simulink model "UAV_modelo_naolinear_2"  (R2017a)
settings: Solver=ode45  StartTime=0.0  StopTime=T_sim  RelTol=1e-3  EnableMultiTasking=on
InitFcn:
  | main
values from neighbouring files (symbols this model uses):
  g = 9.8    [main_model1.m]    (also in main_model2.m; main_modelo_linear_v1.m; main_modelo_linear_v2.m; main_modelo_nao_linear_v1.m)
  incluir_din_motor = -1    [main_model1.m]    (also in main_model2.m; main_modelo_nao_linear_v1.m = 1; main_modelo_nao_linear_v2.m; modelo_naolinear.m = 1)
  Ir = 1e-3    (= 0.001)    [main_model1.m]    (also in main_model2.m; main_modelo_linear_v1.m = 0.01; main_modelo_linear_v2.m = 0.01; main_modelo_nao_linear_v1.m)
  Ixx = 1e-2    (= 0.01)    [main_model1.m]    (also in main_model2.m; main_modelo_linear_v1.m; main_modelo_linear_v2.m; main_modelo_nao_linear_v1.m)
  Iyy = 1e-2    (= 0.01)    [main_model1.m]    (also in main_model2.m; main_modelo_linear_v1.m; main_modelo_linear_v2.m; main_modelo_nao_linear_v1.m)
  Izz = 1.8e-2    (= 0.018)    [main_model1.m]    (also in main_model2.m; main_modelo_linear_v1.m; main_modelo_linear_v2.m; main_modelo_nao_linear_v1.m)
  K = are(A22, B22*inv(R)*B22',C'*Q*C)    [modelo_naolinear.m]    (also in modelo_naolinear_params.m)
  Kd_rot = 0.01    [main_model1.m]    (also in main_model2.m; main_modelo_linear_v1.m = 0; main_modelo_linear_v2.m = 0; main_modelo_nao_linear_v1.m)
  Kd_trans = 0.002    [main_model1.m]    (also in main_model2.m = -0.13723; main_modelo_linear_v1.m = 0; main_modelo_linear_v2.m = 0; main_modelo_nao_linear_v1.m)
  Ki_rot = 1.0    (= 1)    [main_model1.m]    (also in main_model2.m; main_modelo_linear_v1.m = 0.5; main_modelo_linear_v2.m = 0.5; main_modelo_nao_linear_v1.m)
  Ki_trans = 0.06    [main_model1.m]    (also in main_model2.m = 0.41774; main_modelo_linear_v1.m = 0; main_modelo_linear_v2.m = 1; main_modelo_nao_linear_v1.m)
  Kp = 0.9182    [main_model1.m]    (also in main_model2.m; main_modelo_nao_linear_v1.m; main_modelo_nao_linear_v2.m; modelo_naolinear.m)
  Kp_rot = 10    [main_model1.m]    (also in main_model2.m; main_modelo_linear_v1.m = 1; main_modelo_linear_v2.m = 1; main_modelo_nao_linear_v1.m)
  Kp_trans = 0.4    [main_model1.m]    (also in main_model2.m = 2.0968; main_modelo_linear_v1.m = 1; main_modelo_linear_v2.m = 2; main_modelo_nao_linear_v1.m)
  m = 1.0428    [main_model1.m]    (also in main_model2.m; main_modelo_linear_v1.m = 1; main_modelo_linear_v2.m = 1; main_modelo_nao_linear_v1.m)
  N_rot = 100    [main_model2.m]    (also in main_modelo_nao_linear_v2.m; modelo_naolinear.m; modelo_naolinear_params.m)
  N_trans = 5.5815    [main_model2.m]    (also in main_modelo_nao_linear_v2.m; modelo_naolinear.m; modelo_naolinear_params.m)
  p0 = 0    [main_model2.m]    (also in main_modelo_linear_v1.m; main_modelo_linear_v2.m; main_modelo_nao_linear_v2.m; modelo_naolinear.m)
  phi0 = 0    [main_model1.m]    (also in main_model2.m; main_modelo_linear_v1.m; main_modelo_linear_v2.m; main_modelo_nao_linear_v1.m)
  psi0 = 0    [main_model1.m]    (also in main_model2.m; main_modelo_linear_v1.m; main_modelo_linear_v2.m; main_modelo_nao_linear_v1.m)
  q0 = 0    [main_model2.m]    (also in main_modelo_linear_v1.m; main_modelo_linear_v2.m; main_modelo_nao_linear_v2.m; modelo_naolinear.m)
  r0 = 0    [main_model2.m]    (also in main_modelo_linear_v1.m; main_modelo_linear_v2.m; main_modelo_nao_linear_v2.m; modelo_naolinear.m)
  select_controlador = -1    [main_model2.m]    (also in main_modelo_nao_linear_v2.m)
  T = [kf,kf,kf,kf ... (first row only)    [main_model1.m]    (also in main_model2.m; main_modelo_nao_linear_v1.m; main_modelo_nao_linear_v2.m; modelo_naolinear.m)
  T_inv = T^(-1)    [main_model1.m]    (also in main_model2.m; main_modelo_nao_linear_v1.m; main_modelo_nao_linear_v2.m; modelo_naolinear.m)
  tau_a = 0.0569    [main_model1.m]    (also in main_model2.m; main_modelo_nao_linear_v1.m; main_modelo_nao_linear_v2.m; modelo_naolinear.m)
  tau_s = 0.0452    [main_model1.m]    (also in main_model2.m; main_modelo_nao_linear_v1.m; main_modelo_nao_linear_v2.m; modelo_naolinear.m)
  theta0 = 0    [main_model1.m]    (also in main_model2.m; main_modelo_linear_v1.m; main_modelo_linear_v2.m; main_modelo_nao_linear_v1.m)
  vx0 = 0    [main_model1.m]    (also in main_model2.m; main_modelo_nao_linear_v1.m; main_modelo_nao_linear_v2.m; modelo_naolinear.m)
  vxd = 0    [main_model1.m]    (also in main_model2.m; main_modelo_linear_v1.m; main_modelo_linear_v2.m; main_modelo_nao_linear_v1.m)
  vy0 = 0    [main_model1.m]    (also in main_model2.m; main_modelo_nao_linear_v1.m; main_modelo_nao_linear_v2.m; modelo_naolinear.m)
  vyd = 0    [main_model1.m]    (also in main_model2.m; main_modelo_linear_v1.m; main_modelo_linear_v2.m; main_modelo_nao_linear_v1.m)
  vz0 = 0    [main_model1.m]    (also in main_model2.m; main_modelo_nao_linear_v1.m; main_modelo_nao_linear_v2.m; modelo_naolinear.m)
  x0 = 0    [main_model1.m]    (also in main_model2.m; main_modelo_linear_v1.m; main_modelo_linear_v2.m; main_modelo_nao_linear_v1.m)
  y0 = 0    [main_model1.m]    (also in main_model2.m; main_modelo_linear_v1.m; main_modelo_linear_v2.m; main_modelo_nao_linear_v1.m)
  z0 = 1    [main_model1.m]    (also in main_model2.m; main_modelo_linear_v1.m; main_modelo_linear_v2.m; main_modelo_nao_linear_v1.m)
undefined symbols (not defined in the file or in its folder): sigbuilder_block
libraries: simulink x6
settings Model: Creator=dferr  LastModifiedBy=diego
settings DataIOCC: LimitDataPoints=on  SaveFormat=Array
settings OptimizationCC: LifeSpan=inf
settings DebuggingCC: SFUnexpectedBacktrackingDiag=warning  SFNoUnconditionalDefaultTransitionDiag=warning  SFExecutionAtInitializationDiag=none
settings HardwareCC: ProdBitPerPointer=32  ProdBitPerSizeT=32  ProdBitPerPtrDiffT=32  ProdLargestAtomicFloat=None  ProdIntDivRoundTo=Undefined  ProdEndianess=Unspecified  ProdWordSize=32  ProdHWDeviceType=32-bit Generic
settings ModelReferenceCC: PropagateSignalLabelsOutOfModel=off
settings GRTTargetCC: TargetLangStandard=C89/C90 (ANSI)  GeneratePreprocessorConditionals=Disable all
settings ConfigComp: CovMetricSettings=dw  CovHtmlReporting=on  CovSaveCumulativeToWorkspaceVar=on  CovSaveSingleToWorkspaceVar=on  CovExternalEMLEnable=off  CovSFcnEnable=off

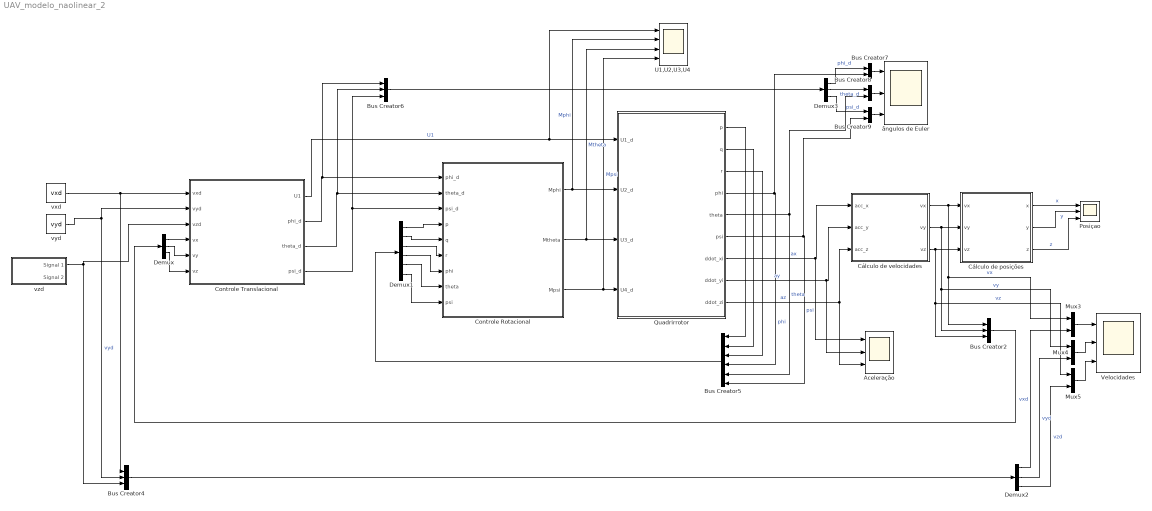
== system UAV_modelo_naolinear_2 ==
  Aceleração : Scope  NumInputPorts=3
  Bus Creator2 : BusCreator  Inputs=3
  Bus Creator4 : BusCreator  Inputs=3
  Bus Creator5 : BusCreator  Inputs=6
  Bus Creator6 : BusCreator  Inputs=3
  Bus Creator7 : BusCreator  Inputs=2
  Bus Creator8 : BusCreator  Inputs=2
  Bus Creator9 : BusCreator  Inputs=2
  Controle Rotacional : Subsystem
      mask Display:
      | disp('Controle Rotacional')
      | port_label('input',1,'phi_d')
      | port_label('input',2,'theta_d')
      | port_label('input',3,'psi_d')
      | port_label('input',4,'p')
      | port_label('input',5,'q')
      | port_label('input',6,'r')
      | port_label('input',7,'phi')
      | port_label('input',8,'theta')
      | port_label('input',9,'psi')
      | port_label('output',1,'Mphi')
      | port_label('output',2,'Mtheta')
      | port_label('output',3,'Mpsi')
  Controle Translacional : Subsystem
      mask Display:
      | disp('Controle Translacional')
      | port_label('input',1,'vxd')
      | port_label('input',2,'vyd')
      | port_label('input',3,'vzd')
      | port_label('input',4,'vx')
      | port_label('input',5,'vy')
      | port_label('input',6,'vz')
      | port_label('output',1,'U1')
      | port_label('output',2,'phi_d')
      | port_label('output',3,'theta_d')
      | port_label('output',4,'psi_d')
  Cálculo de posições : Subsystem
      mask Display:
      | disp('Vel -> Pos')
      | port_label('input',1,'vel_x')
      | port_label('input',2,'vel_y')
      | port_label('input',3,'vel_ z')
      | port_label('output',1,'x')
      | port_label('output',2,'y')
      | port_label('output',3,'z')
  Cálculo de velocidades : Subsystem
      mask Display:
      | disp('Acc -> Vel')
      | port_label('input',1,'acc_x')
      | port_label('input',2,'acc_y')
      | port_label('input',3,'acc_z')
      | port_label('output',1,'vel_x')
      | port_label('output',2,'vel_y')
      | port_label('output',3,'vel_z')
  Demux : Demux  Outputs=3
  Demux1 : Demux  Outputs=6
  Demux2 : Demux  Outputs=3
  Demux3 : Demux  Outputs=3
  Mux3 : Mux  Inputs=2
  Mux4 : Mux  Inputs=2
  Mux5 : Mux  Inputs=2
  Posiçao : Scope  NumInputPorts=3
  Quadrirrotor : Subsystem
      mask Display:
      | disp('Quadrirrotor')
      | port_label('input',1,'U1')
      | port_label('input',2,'U2')
      | port_label('input',3,'U3')
      | port_label('input',4,'U4')
      | port_label('output',1,'p')
      | port_label('output',2,'q')
      | port_label('output',3,'r')
      | port_label('output',4,'phi')
      | port_label('output',5,'theta')
      | port_label('output',6,'psi')
      | port_label('output',7,'ddot_xi')
      | port_label('output',8,'ddot_yi')
      | port_label('output',9,'ddot_zi')
  U1,U2,U3,U4 : Scope  NumInputPorts=4
  Velocidades : Scope  NumInputPorts=3
  vxd : Constant  Value=vxd
  vyd : Constant  Value=vyd
  vzd : Subsystem  Tag=STV Subsys  LoadFcn=sigbuilder_block('load');  StartFcn=sigbuilder_block('start');  StopFcn=sigbuilder_block('stop');  ClipboardFcn=sigbuilder_block('clipboard');  mask(Sigbuilder block){tuvar=[0:10]}
      mask help: Simulink:masks:SigbuilderBlock_MD
      mask init:
      | if ~strcmp(get_param(bdroot(gcbh),'SimulationStatus'),'stopped') tuvar = sigbuilder_block('maskInit'); end
      settings: CopyFcn=sigbuilder_block('copy');  DeleteFcn=sigbuilder_block('delete');  ModelCloseFcn=sigbuilder_block('modelClose');  PreSaveFcn=sigbuilder_block('preSave');  PauseFcn=sigbuilder_block('pause');  ContinueFcn=sigbuilder_block('continue');  NameChangeFcn=sigbuilder_block('namechange');  OpenFcn=sigbuilder_block('open',[437.6 199.2 550.4 400 ]);  CloseFcn=sigbuilder_block('close');
      mask Display: plot(0, 0, 100, 100,[2, 2, 32, 32, 2], [68, 8, 8, 68, 68],[32, 2], [38, 38], [32, 19, 2],[53, 60, 44], [32, 17, 17, 2],[16, 16, 31, 31]);txt = getActiveGroup(gcbh);text(2, 100, txt,'verticalAlignment', 'top');
  ângulos de Euler : Scope  NumInputPorts=3
  wires:
  Cálculo de velocidades/1(vx) -> Mux3/1, Bus Creator2/1, Cálculo de posições/1(vx)  "vx"
  Cálculo de velocidades/2(vy) -> Mux4/1, Bus Creator2/2, Cálculo de posições/2(vy)  "vy"
  Cálculo de velocidades/3(vz) -> Mux5/1, Bus Creator2/3, Cálculo de posições/3(vz)  "vz"
  Bus Creator2/1 -> Demux/1
  vyd/1 -> Controle Translacional/2(vyd), Bus Creator4/2  "vyd"
  Demux1/1 -> Controle Rotacional/4(p)
  Demux1/2 -> Controle Rotacional/5(q)
  Demux1/3 -> Controle Rotacional/6(r)
  Demux1/4 -> Controle Rotacional/7(phi)
  Demux1/5 -> Controle Rotacional/8(theta)
  Demux1/6 -> Controle Rotacional/9(psi)
  Bus Creator5/1 -> Demux1/1
  Mux3/1 -> Velocidades/1
  Mux4/1 -> Velocidades/2
  Mux5/1 -> Velocidades/3
  Bus Creator4/1 -> Demux2/1
  Demux2/1 -> Mux3/2  "vxd"
  Demux2/2 -> Mux4/2  "vyd"
  Demux2/3 -> Mux5/2  "vzd"
  Controle Rotacional/1(Mphi) -> U1,U2,U3,U4/2, Quadrirrotor/2(U2_d)  "Mphi"
  Controle Rotacional/2(Mtheta) -> U1,U2,U3,U4/3, Quadrirrotor/3(U3_d)  "Mtheta"
  Controle Rotacional/3(Mpsi) -> U1,U2,U3,U4/4, Quadrirrotor/4(U4_d)  "Mpsi"
  Quadrirrotor/1(p) -> Bus Creator5/1
  Quadrirrotor/2(q) -> Bus Creator5/2
  Quadrirrotor/3(r) -> Bus Creator5/3
  Quadrirrotor/4(phi) -> Bus Creator7/2, Bus Creator5/4  "phi"
  Quadrirrotor/5(theta) -> Bus Creator5/5, Bus Creator8/2  "theta"
  Quadrirrotor/6(psi) -> Bus Creator9/2, Bus Creator5/6  "psi"
  Quadrirrotor/7(ddot_xi) -> Aceleração/1, Cálculo de velocidades/1(acc_x)  "ax"
  Quadrirrotor/8(ddot_yi) -> Aceleração/2, Cálculo de velocidades/2(acc_y)  "ay"
  Quadrirrotor/9(ddot_zi) -> Aceleração/3, Cálculo de velocidades/3(acc_z)  "az"
  Demux/1 -> Controle Translacional/4(vx)
  Demux/2 -> Controle Translacional/5(vy)
  Demux/3 -> Controle Translacional/6(vz)
  Controle Translacional/1(U1) -> U1,U2,U3,U4/1, Quadrirrotor/1(U1_d)  "U1"
  Controle Translacional/2(phi_d) -> Bus Creator6/1, Controle Rotacional/1(phi_d)
  Controle Translacional/3(theta_d) -> Bus Creator6/2, Controle Rotacional/2(theta_d)
  Controle Translacional/4(psi_d) -> Bus Creator6/3, Controle Rotacional/3(psi_d)
  Bus Creator6/1 -> Demux3/1
  Bus Creator7/1 -> ângulos de Euler/1
  Bus Creator8/1 -> ângulos de Euler/2
  Bus Creator9/1 -> ângulos de Euler/3
  Demux3/1 -> Bus Creator7/1  "phi_d"
  Demux3/2 -> Bus Creator8/1  "theta_d"
  Demux3/3 -> Bus Creator9/1  "psi_d"
  vxd/1 -> Bus Creator4/1, Controle Translacional/1(vxd)
  Cálculo de posições/1(x) -> Posiçao/1  "x"
  Cálculo de posições/2(y) -> Posiçao/2  "y"
  Cálculo de posições/3(z) -> Posiçao/3  "z"
  vzd/1(Signal 1) -> Controle Translacional/3(vzd), Bus Creator4/3

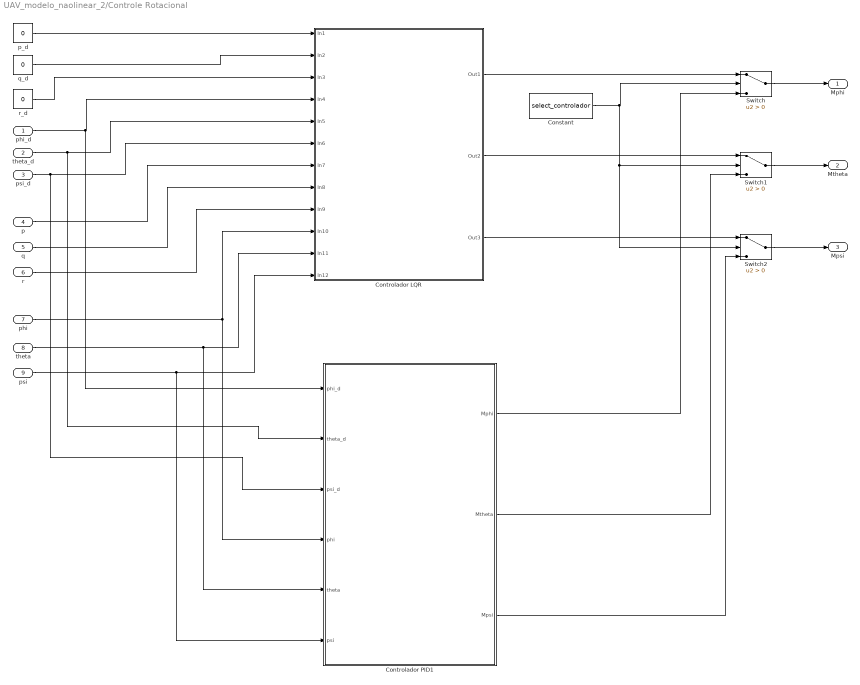
== system UAV_modelo_naolinear_2/Controle Rotacional ==
  phi_d : Inport
  theta_d : Inport  Port=2
  psi_d : Inport  Port=3
  p : Inport  Port=4
  q : Inport  Port=5
  r : Inport  Port=6
  phi : Inport  Port=7
  theta : Inport  Port=8
  psi : Inport  Port=9
  Constant : Constant  Value=select_controlador
  Controlador LQR : Subsystem
      mask Display:
      | disp('Controlador LQR')
      | port_label('input',1,'p_d')
      | port_label('input',2,'q_d')
      | port_label('input',3,'r_d')
      | port_label('input',4,'phi_d')
      | port_label('input',5,'theta_d')
      | port_label('input',6,'psi_d')
      | port_label('input',7,'p')
      | port_label('input',8,'q')
      | port_label('input',9,'r')
      | port_label('input',10,'phi')
      | port_label('input',11,'theta')
      | port_label('input',12,'psi')
      | port_label('output',1,'Mphi')
      | port_label('output',2,'Mtheta')
      | port_label('output',3,'Mpsi')
  Controlador PID1 : Subsystem
      mask Display:
      | disp('Controlador PID')
      | port_label('input',1,'phi_d')
      | port_label('input',2,'theta_d')
      | port_label('input',3,'psi_d')
      | port_label('input',4,'phi')
      | port_label('input',5,'theta')
      | port_label('input',6,'psi')
      | port_label('output',1,'Mphi')
      | port_label('output',2,'Mtheta')
      | port_label('output',3,'Mpsi')
  Switch : Switch  Criteria=u2 > Threshold
  Switch1 : Switch  Criteria=u2 > Threshold
  Switch2 : Switch  Criteria=u2 > Threshold
  p_d : Constant  Value=0
  q_d : Constant  Value=0
  r_d : Constant  Value=0
  Mphi : Outport
  Mtheta : Outport  Port=2
  Mpsi : Outport  Port=3
  wires:
  p_d/1 -> Controlador LQR/1(In1)
  q_d/1 -> Controlador LQR/2(In2)
  r_d/1 -> Controlador LQR/3(In3)
  phi_d/1 -> Controlador PID1/1(phi_d), Controlador LQR/4(In4)
  theta_d/1 -> Controlador PID1/2(theta_d), Controlador LQR/5(In5)
  psi_d/1 -> Controlador PID1/3(psi_d), Controlador LQR/6(In6)
  p/1 -> Controlador LQR/7(In7)
  q/1 -> Controlador LQR/8(In8)
  r/1 -> Controlador LQR/9(In9)
  phi/1 -> Controlador PID1/4(phi), Controlador LQR/10(In10)
  theta/1 -> Controlador PID1/5(theta), Controlador LQR/11(In11)
  psi/1 -> Controlador PID1/6(psi), Controlador LQR/12(In12)
  Controlador LQR/1(Out1) -> Switch/1
  Controlador LQR/3(Out3) -> Switch2/1
  Controlador LQR/2(Out2) -> Switch1/1
  Switch/1 -> Mphi/1
  Switch1/1 -> Mtheta/1
  Switch2/1 -> Mpsi/1
  Constant/1 -> Switch2/2, Switch1/2, Switch/2
  Controlador PID1/1(Mphi) -> Switch/3
  Controlador PID1/2(Mtheta) -> Switch1/3
  Controlador PID1/3(Mpsi) -> Switch2/3

== system UAV_modelo_naolinear_2/Controle Translacional ==
  vxd : Inport
  vyd : Inport  Port=2
  vzd : Inport  Port=3
  vx : Inport  Port=4
  vy : Inport  Port=5
  vz : Inport  Port=6
  Controle de velocidade : Subsystem
      mask Display:
      | disp('Controle de Velocidade PID')
      | port_label('input',1,'vxd')
      | port_label('input',2,'vyd')
      | port_label('input',3,'vzd')
      | port_label('input',4,'vx')
      | port_label('input',5,'vy')
      | port_label('input',6,'vz')
      | 
      | port_label('output',1,'u1')
      | port_label('output',2,'u2')
      | port_label('output',3,'u3')
  Entradas virtuais : Subsystem
      mask Display:
      | disp('(u1,u2,u3)->(eta_d,U1)')
      | port_label('input',1,'u1')
      | port_label('input',2,'u2')
      | port_label('input',3,'u3')
      | port_label('output',1,'phi_d')
      | port_label('output',2,'theta_d')
      | port_label('output',3,'psi_d')
      | port_label('output',4,'U1')
  U1 : Outport
  phi_d : Outport  Port=2
  theta_d : Outport  Port=3
  psi_d : Outport  Port=4
  wires:
  Controle de velocidade/2(u2) -> Entradas virtuais/2(u2)
  Entradas virtuais/1(phi_d) -> phi_d/1  "phi_d"
  Entradas virtuais/2(theta_d) -> theta_d/1  "theta_d"
  Entradas virtuais/3(psi_d) -> psi_d/1  "psi_d"
  Controle de velocidade/1(u1) -> Entradas virtuais/1(u1)
  vz/1 -> Controle de velocidade/6(vz)
  vy/1 -> Controle de velocidade/5("vy ")
  Controle de velocidade/3(u3) -> Entradas virtuais/3(u3)
  vx/1 -> Controle de velocidade/4(vx)
  Entradas virtuais/4(U1) -> U1/1  "Tb"
  vyd/1 -> Controle de velocidade/2(vyd)
  vzd/1 -> Controle de velocidade/3(vzd)
  vxd/1 -> Controle de velocidade/1(vxd)

== system UAV_modelo_naolinear_2/Cálculo de posições ==
  vx : Inport
  vy : Inport  Port=2
  vz : Inport  Port=3
  Integrator : Integrator  InitialCondition=x0
  Integrator1 : Integrator  InitialCondition=y0
  Integrator2 : Integrator  InitialCondition=z0  LimitOutput=on  LowerSaturationLimit=0
  x : Outport
  y : Outport  Port=2
  z : Outport  Port=3
  wires:
  Integrator/1 -> x/1
  Integrator1/1 -> y/1
  vy/1 -> Integrator1/1
  vz/1 -> Integrator2/1
  vx/1 -> Integrator/1
  Integrator2/1 -> z/1

== system UAV_modelo_naolinear_2/Cálculo de velocidades ==
  acc_x : Inport
  acc_y : Inport  Port=2
  acc_z : Inport  Port=3
  Integrator : Integrator  InitialCondition=vx0  ZeroCross=off
  Integrator1 : Integrator  InitialCondition=vy0  ZeroCross=off
  Integrator2 : Integrator  InitialCondition=vz0  ZeroCross=off
  vx : Outport
  vy : Outport  Port=2
  vz : Outport  Port=3
  wires:
  Integrator2/1 -> vz/1
  acc_z/1 -> Integrator2/1
  Integrator/1 -> vx/1
  acc_x/1 -> Integrator/1
  acc_y/1 -> Integrator1/1
  Integrator1/1 -> vy/1

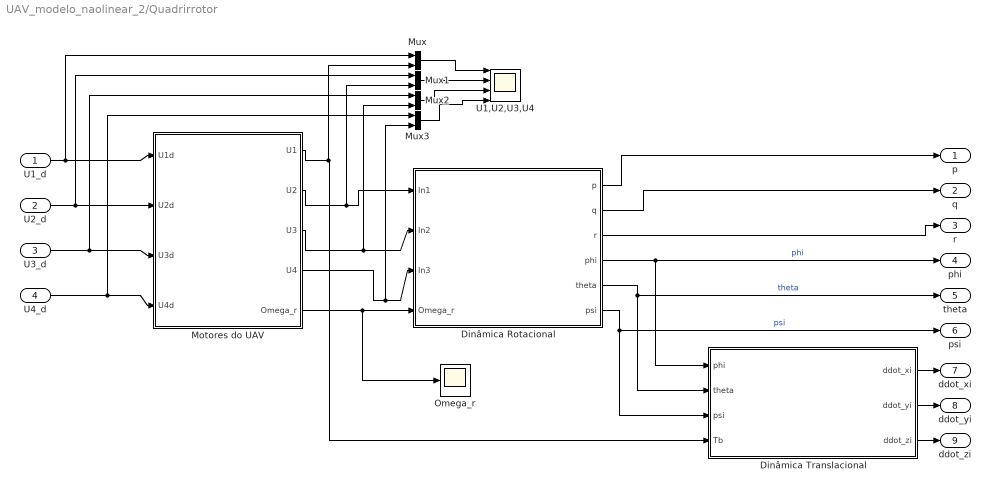
== system UAV_modelo_naolinear_2/Quadrirrotor ==
  U1_d : Inport
  U2_d : Inport  Port=2
  U3_d : Inport  Port=3
  U4_d : Inport  Port=4
  Dinâmica Rotacional : Subsystem
      mask Display:
      | disp('Dinâmica Rotacional')
      | port_label('input',1,'Mphi')
      | port_label('input',2,'Mtheta')
      | port_label('input',3,'Mpsi')
      | port_label('input',4,'Omega_r')
      | port_label('output',1,'p')
      | port_label('output',2,'q')
      | port_label('output',3,'r')
      | port_label('output',4,'phi')
      | port_label('output',5,'theta')
      | port_label('output',6,'psi')
  Dinâmica Translacional : Subsystem
      mask Display:
      | disp ('Dinâmica Translacional')
      | port_label('input',1,'phi')
      | port_label('input',2,'theta')
      | port_label('input',3,'psi')
      | port_label('input',4,'Tb')
      | port_label('output',1,'ddot_xi')
      | port_label('output',2,'ddot_yi')
      | port_label('output',3,'ddot_zi')
  "Motores do UAV " : Subsystem
      mask Display:
      | disp('Dinâmica Motores')
      | port_label('input',1,'U1d')
      | port_label('input',2,'U2d')
      | port_label('input',3,'U3d')
      | port_label('input',4,'U4d')
      | port_label('output',1,'U1')
      | port_label('output',2,'U2')
      | port_label('output',3,'U3')
      | port_label('output',4,'U4')
      | port_label('output',5,'Omega_r')
  Mux{,1..3} (4 alike) : Mux  Inputs=2
  Omega_r : Scope
  U1,U2,U3,U4 : Scope  NumInputPorts=4
  p : Outport
  q : Outport  Port=2
  r : Outport  Port=3
  phi : Outport  Port=4
  theta : Outport  Port=5
  psi : Outport  Port=6
  ddot_xi : Outport  Port=7
  ddot_yi : Outport  Port=8
  ddot_zi : Outport  Port=9
  wires:
  Dinâmica Rotacional/6(psi) -> psi/1, Dinâmica Translacional/3(psi)  "psi"
  Dinâmica Rotacional/5(theta) -> theta/1, Dinâmica Translacional/2(theta)  "theta"
  Dinâmica Rotacional/4(phi) -> Dinâmica Translacional/1(phi), phi/1  "phi"
  Dinâmica Rotacional/1(p) -> p/1
  Dinâmica Rotacional/2(q) -> q/1
  Dinâmica Rotacional/3(r) -> r/1
  Dinâmica Translacional/1(ddot_xi) -> ddot_xi/1
  Dinâmica Translacional/2(ddot_yi) -> ddot_yi/1
  Dinâmica Translacional/3(ddot_zi) -> ddot_zi/1
  U2_d/1 -> "Motores do UAV "/2(U2d), Mux1/1
  U3_d/1 -> "Motores do UAV "/3(U3d), Mux2/1
  Mux/1 -> U1,U2,U3,U4/1
  Mux1/1 -> U1,U2,U3,U4/2
  Mux2/1 -> U1,U2,U3,U4/3
  Mux3/1 -> U1,U2,U3,U4/4
  "Motores do UAV "/3(U3) -> Mux2/2, Dinâmica Rotacional/2(In2)
  "Motores do UAV "/4(U4) -> Mux3/2, Dinâmica Rotacional/3(In3)
  "Motores do UAV "/2(U2) -> Mux1/2, Dinâmica Rotacional/1(In1)
  "Motores do UAV "/1(U1) -> Mux/2, Dinâmica Translacional/4(Tb)
  U1_d/1 -> "Motores do UAV "/1(U1d), Mux/1
  U4_d/1 -> "Motores do UAV "/4(U4d), Mux3/1
  "Motores do UAV "/5(Omega_r) -> Omega_r/1, Dinâmica Rotacional/4(Omega_r)

== system UAV_modelo_naolinear_2/vzd ==
  Demux : Demux  Tag=STV Demux  Outputs=2
  FromWs : FromWorkspace  Tag=STV FromWs  VariableName=tuvar  SampleTime=0
      SigBuilderData=|
      | common.afterFinalStr = 'Extrapolate'
      | common.sampleTime = 0
      | dataSet.timeRange = [0 20]
      | dataSet.name = 'Group 1'
      | sbobj.Groups.Name = 'Group 1'
      | sbobj.Groups.Signals(1).Name = 'Signal 1'
      | sbobj.Groups.Signals(1).XData = [0 2.05 4.75 8 18 20]
      | sbobj.Groups.Signals(1).YData = [-0.2 8.5 20 20 0 0]
      | sbobj.Groups.Signals(2).Name = 'Signal 2'
      | sbobj.Groups.Signals(2).XData = [0 5 5 20]
      | sbobj.Groups.Signals(2).YData = [0 0 1 1]
      | sbobj.Groups.TimeRange = [0 20]
  Signal 1 : Outport  Tag=STV Outport
  Signal 2 : Outport  Tag=STV Outport  Port=2
  wires:
  FromWs/1 -> Demux/1
  Demux/1 -> Signal 1/1
  Demux/2 -> Signal 2/1

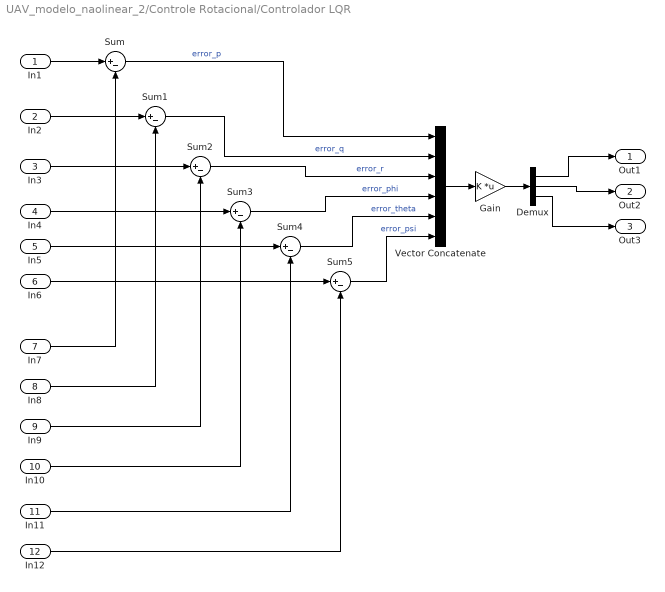
== system UAV_modelo_naolinear_2/Controle Rotacional/Controlador LQR ==
  In1 : Inport
  In2 : Inport  Port=2
  In3 : Inport  Port=3
  In4 : Inport  Port=4
  In5 : Inport  Port=5
  In6 : Inport  Port=6
  In7 : Inport  Port=7
  In8 : Inport  Port=8
  In9 : Inport  Port=9
  In10 : Inport  Port=10
  In11 : Inport  Port=11
  In12 : Inport  Port=12
  Demux : Demux  Outputs=3
  Gain : Gain  Gain=K  Multiplication=Matrix(K*u)
  Sum{,1..5} (6 alike) : Sum  Inputs=|+-
  Vector Concatenate : Concatenate  NumInputs=6
  Out1 : Outport
  Out2 : Outport  Port=2
  Out3 : Outport  Port=3
  wires:
  In3/1 -> Sum2/1
  Sum4/1 -> Vector Concatenate/5  "error_theta"
  Gain/1 -> Demux/1
  Demux/2 -> Out2/1
  In5/1 -> Sum4/1
  In11/1 -> Sum4/2
  Demux/3 -> Out3/1
  In4/1 -> Sum3/1
  Vector Concatenate/1 -> Gain/1
  Sum5/1 -> Vector Concatenate/6  "error_psi"
  In8/1 -> Sum1/2
  In2/1 -> Sum1/1
  In1/1 -> Sum/1
  In12/1 -> Sum5/2
  In9/1 -> Sum2/2
  Demux/1 -> Out1/1
  Sum2/1 -> Vector Concatenate/3  "error_r"
  In6/1 -> Sum5/1
  In7/1 -> Sum/2
  In10/1 -> Sum3/2
  Sum/1 -> Vector Concatenate/1  "error_p"
  Sum1/1 -> Vector Concatenate/2  "error_q"
  Sum3/1 -> Vector Concatenate/4  "error_phi"

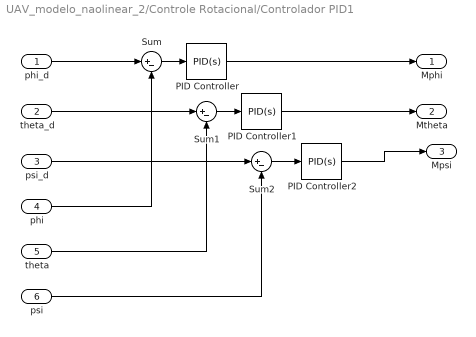
== system UAV_modelo_naolinear_2/Controle Rotacional/Controlador PID1 ==
  phi_d : Inport
  theta_d : Inport  Port=2
  psi_d : Inport  Port=3
  phi : Inport  Port=4
  theta : Inport  Port=5
  psi : Inport  Port=6
  PID Controller : simulink/Continuous/PID Controller  Controller=PID  TimeDomain=Continuous-time  SampleTime=-1  IntegratorMethod=Forward Euler  FilterMethod=Forward Euler  Form=Ideal  UseFilter=on  ControllerParametersSource=internal  P=Kp_rot  I=Ki_rot  D=Kd_rot  N=N_rot  InitialConditionSource=internal  InitialConditionForIntegrator=0  InitialConditionForFilter=0  ExternalReset=none  LimitOutput=off  UpperSaturationLimit=inf  LowerSaturationLimit=-inf  LinearizeAsGain=on  AntiWindupMode=none  Kb=1  TrackingMode=off  Kt=1  PParamMin=[]  PParamMax=[]  IParamMin=[]  IParamMax=[]  DParamMin=[]  DParamMax=[]  NParamMin=[]  NParamMax=[]  KbParamMin=[]  KbParamMax=[]  KtParamMin=[]  KtParamMax=[]  POutMin=[]  POutMax=[]  IOutMin=[]  IOutMax=[]  DOutMin=[]  DOutMax=[]  NOutMin=[]  NOutMax=[]  KbOutMin=[]  KbOutMax=[]  KtOutMin=[]  KtOutMax=[]  IntegratorOutMin=[]  IntegratorOutMax=[]  FilterOutMin=[]  FilterOutMax=[]  SumOutMin=[]  SumOutMax=[]  SumI1OutMin=[]  SumI1OutMax=[]  SumI2OutMin=[]  SumI2OutMax=[]  SumI3OutMin=[]  SumI3OutMax=[]  SumDOutMin=[]  SumDOutMax=[]  SaturationOutMin=[]  SaturationOutMax=[]  IntegratorContinuousStateAttributes=''  IntegratorStateMustResolveToSignalObject=off  IntegratorRTWStateStorageClass=Auto  FilterContinuousStateAttributes=''  FilterStateMustResolveToSignalObject=off  FilterRTWStateStorageClass=Auto  DifferentiatorICPrevScaledInput=0  DifferentiatorOutMin=[]  DifferentiatorOutMax=[]  InitialConditionSetting=State (most efficient)
  PID Controller1 : simulink/Continuous/PID Controller  Controller=PID  TimeDomain=Continuous-time  SampleTime=-1  IntegratorMethod=Forward Euler  FilterMethod=Forward Euler  Form=Ideal  UseFilter=on  ControllerParametersSource=internal  P=Kp_rot  I=Ki_rot  D=Kd_rot  N=N_rot  InitialConditionSource=internal  InitialConditionForIntegrator=0  InitialConditionForFilter=0  ExternalReset=none  LimitOutput=off  UpperSaturationLimit=inf  LowerSaturationLimit=-inf  LinearizeAsGain=on  AntiWindupMode=none  Kb=1  TrackingMode=off  Kt=1  PParamMin=[]  PParamMax=[]  IParamMin=[]  IParamMax=[]  DParamMin=[]  DParamMax=[]  NParamMin=[]  NParamMax=[]  KbParamMin=[]  KbParamMax=[]  KtParamMin=[]  KtParamMax=[]  POutMin=[]  POutMax=[]  IOutMin=[]  IOutMax=[]  DOutMin=[]  DOutMax=[]  NOutMin=[]  NOutMax=[]  KbOutMin=[]  KbOutMax=[]  KtOutMin=[]  KtOutMax=[]  IntegratorOutMin=[]  IntegratorOutMax=[]  FilterOutMin=[]  FilterOutMax=[]  SumOutMin=[]  SumOutMax=[]  SumI1OutMin=[]  SumI1OutMax=[]  SumI2OutMin=[]  SumI2OutMax=[]  SumI3OutMin=[]  SumI3OutMax=[]  SumDOutMin=[]  SumDOutMax=[]  SaturationOutMin=[]  SaturationOutMax=[]  IntegratorContinuousStateAttributes=''  IntegratorStateMustResolveToSignalObject=off  IntegratorRTWStateStorageClass=Auto  FilterContinuousStateAttributes=''  FilterStateMustResolveToSignalObject=off  FilterRTWStateStorageClass=Auto  DifferentiatorICPrevScaledInput=0  DifferentiatorOutMin=[]  DifferentiatorOutMax=[]  InitialConditionSetting=State (most efficient)
  PID Controller2 : simulink/Continuous/PID Controller  Controller=PID  TimeDomain=Continuous-time  SampleTime=-1  IntegratorMethod=Forward Euler  FilterMethod=Forward Euler  Form=Ideal  UseFilter=on  ControllerParametersSource=internal  P=Kp_rot  I=Ki_rot  D=Kd_rot  N=N_rot  InitialConditionSource=internal  InitialConditionForIntegrator=0  InitialConditionForFilter=0  ExternalReset=none  LimitOutput=off  UpperSaturationLimit=inf  LowerSaturationLimit=-inf  LinearizeAsGain=on  AntiWindupMode=none  Kb=1  TrackingMode=off  Kt=1  PParamMin=[]  PParamMax=[]  IParamMin=[]  IParamMax=[]  DParamMin=[]  DParamMax=[]  NParamMin=[]  NParamMax=[]  KbParamMin=[]  KbParamMax=[]  KtParamMin=[]  KtParamMax=[]  POutMin=[]  POutMax=[]  IOutMin=[]  IOutMax=[]  DOutMin=[]  DOutMax=[]  NOutMin=[]  NOutMax=[]  KbOutMin=[]  KbOutMax=[]  KtOutMin=[]  KtOutMax=[]  IntegratorOutMin=[]  IntegratorOutMax=[]  FilterOutMin=[]  FilterOutMax=[]  SumOutMin=[]  SumOutMax=[]  SumI1OutMin=[]  SumI1OutMax=[]  SumI2OutMin=[]  SumI2OutMax=[]  SumI3OutMin=[]  SumI3OutMax=[]  SumDOutMin=[]  SumDOutMax=[]  SaturationOutMin=[]  SaturationOutMax=[]  IntegratorContinuousStateAttributes=''  IntegratorStateMustResolveToSignalObject=off  IntegratorRTWStateStorageClass=Auto  FilterContinuousStateAttributes=''  FilterStateMustResolveToSignalObject=off  FilterRTWStateStorageClass=Auto  DifferentiatorICPrevScaledInput=0  DifferentiatorOutMin=[]  DifferentiatorOutMax=[]  InitialConditionSetting=State (most efficient)
  Sum : Sum  Inputs=|+-
  Sum1 : Sum  Inputs=|+-
  Sum2 : Sum  Inputs=|+-
  Mphi : Outport
  Mtheta : Outport  Port=2
  Mpsi : Outport  Port=3
  wires:
  PID Controller2/1 -> Mpsi/1
  PID Controller1/1 -> Mtheta/1
  PID Controller/1 -> Mphi/1
  Sum/1 -> PID Controller/1
  Sum1/1 -> PID Controller1/1
  Sum2/1 -> PID Controller2/1
  phi_d/1 -> Sum/1
  theta_d/1 -> Sum1/1
  psi_d/1 -> Sum2/1
  phi/1 -> Sum/2
  theta/1 -> Sum1/2
  psi/1 -> Sum2/2

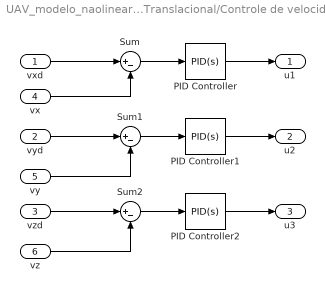
== system UAV_modelo_naolinear_2/Controle Translacional/Controle de velocidade ==
  vxd : Inport
  vyd : Inport  Port=2
  vzd : Inport  Port=3
  vx : Inport  Port=4
  "vy " : Inport  Port=5
  vz : Inport  Port=6
  PID Controller : simulink/Continuous/PID Controller  Controller=PID  TimeDomain=Continuous-time  SampleTime=-1  IntegratorMethod=Forward Euler  FilterMethod=Forward Euler  Form=Parallel  UseFilter=on  ControllerParametersSource=internal  P=Kp_trans  I=Ki_trans  D=Kd_trans  N=N_trans  InitialConditionSource=internal  InitialConditionForIntegrator=0  InitialConditionForFilter=0  ExternalReset=none  LimitOutput=off  UpperSaturationLimit=inf  LowerSaturationLimit=-inf  LinearizeAsGain=on  AntiWindupMode=none  Kb=1  TrackingMode=off  Kt=1  RndMeth=Nearest  PParamMin=[]  PParamMax=[]  IParamMin=[]  IParamMax=[]  DParamMin=[]  DParamMax=[]  NParamMin=[]  NParamMax=[]  KbParamMin=[]  KbParamMax=[]  KtParamMin=[]  KtParamMax=[]  POutMin=[]  POutMax=[]  IOutMin=[]  IOutMax=[]  DOutMin=[]  DOutMax=[]  NOutMin=[]  NOutMax=[]  KbOutMin=[]  KbOutMax=[]  KtOutMin=[]  KtOutMax=[]  IntegratorOutMin=[]  IntegratorOutMax=[]  FilterOutMin=[]  FilterOutMax=[]  SumOutMin=[]  SumOutMax=[]  SumI1OutMin=[]  SumI1OutMax=[]  SumI2OutMin=[]  SumI2OutMax=[]  SumI3OutMin=[]  SumI3OutMax=[]  SumDOutMin=[]  SumDOutMax=[]  SaturationOutMin=[]  SaturationOutMax=[]  IntegratorContinuousStateAttributes=''  IntegratorStateMustResolveToSignalObject=off  IntegratorRTWStateStorageClass=Auto  FilterContinuousStateAttributes=''  FilterStateMustResolveToSignalObject=off  FilterRTWStateStorageClass=Auto  DifferentiatorICPrevScaledInput=0  DifferentiatorOutMin=[]  DifferentiatorOutMax=[]  InitialConditionSetting=State (most efficient)
      settings: LockScale=on
  PID Controller1 : simulink/Continuous/PID Controller  Controller=PID  TimeDomain=Continuous-time  SampleTime=-1  IntegratorMethod=Forward Euler  FilterMethod=Forward Euler  Form=Parallel  UseFilter=on  ControllerParametersSource=internal  P=Kp_trans  I=Ki_trans  D=Kd_trans  N=100  InitialConditionSource=internal  InitialConditionForIntegrator=0  InitialConditionForFilter=0  ExternalReset=none  LimitOutput=off  UpperSaturationLimit=inf  LowerSaturationLimit=-inf  LinearizeAsGain=on  AntiWindupMode=none  Kb=1  TrackingMode=off  Kt=1  RndMeth=Nearest  PParamMin=[]  PParamMax=[]  IParamMin=[]  IParamMax=[]  DParamMin=[]  DParamMax=[]  NParamMin=[]  NParamMax=[]  KbParamMin=[]  KbParamMax=[]  KtParamMin=[]  KtParamMax=[]  POutMin=[]  POutMax=[]  IOutMin=[]  IOutMax=[]  DOutMin=[]  DOutMax=[]  NOutMin=[]  NOutMax=[]  KbOutMin=[]  KbOutMax=[]  KtOutMin=[]  KtOutMax=[]  IntegratorOutMin=[]  IntegratorOutMax=[]  FilterOutMin=[]  FilterOutMax=[]  SumOutMin=[]  SumOutMax=[]  SumI1OutMin=[]  SumI1OutMax=[]  SumI2OutMin=[]  SumI2OutMax=[]  SumI3OutMin=[]  SumI3OutMax=[]  SumDOutMin=[]  SumDOutMax=[]  SaturationOutMin=[]  SaturationOutMax=[]  IntegratorContinuousStateAttributes=''  IntegratorStateMustResolveToSignalObject=off  IntegratorRTWStateStorageClass=Auto  FilterContinuousStateAttributes=''  FilterStateMustResolveToSignalObject=off  FilterRTWStateStorageClass=Auto  DifferentiatorICPrevScaledInput=0  DifferentiatorOutMin=[]  DifferentiatorOutMax=[]  InitialConditionSetting=State (most efficient)
      settings: LockScale=on
  PID Controller2 : simulink/Continuous/PID Controller  Controller=PID  TimeDomain=Continuous-time  SampleTime=-1  IntegratorMethod=Forward Euler  FilterMethod=Forward Euler  Form=Parallel  UseFilter=on  ControllerParametersSource=internal  P=Kp_trans  I=Ki_trans  D=Kd_trans  N=100  InitialConditionSource=internal  InitialConditionForIntegrator=0  InitialConditionForFilter=0  ExternalReset=none  LimitOutput=off  UpperSaturationLimit=inf  LowerSaturationLimit=-inf  LinearizeAsGain=on  AntiWindupMode=none  Kb=1  TrackingMode=off  Kt=1  RndMeth=Nearest  PParamMin=[]  PParamMax=[]  IParamMin=[]  IParamMax=[]  DParamMin=[]  DParamMax=[]  NParamMin=[]  NParamMax=[]  KbParamMin=[]  KbParamMax=[]  KtParamMin=[]  KtParamMax=[]  POutMin=[]  POutMax=[]  IOutMin=[]  IOutMax=[]  DOutMin=[]  DOutMax=[]  NOutMin=[]  NOutMax=[]  KbOutMin=[]  KbOutMax=[]  KtOutMin=[]  KtOutMax=[]  IntegratorOutMin=[]  IntegratorOutMax=[]  FilterOutMin=[]  FilterOutMax=[]  SumOutMin=[]  SumOutMax=[]  SumI1OutMin=[]  SumI1OutMax=[]  SumI2OutMin=[]  SumI2OutMax=[]  SumI3OutMin=[]  SumI3OutMax=[]  SumDOutMin=[]  SumDOutMax=[]  SaturationOutMin=[]  SaturationOutMax=[]  IntegratorContinuousStateAttributes=''  IntegratorStateMustResolveToSignalObject=off  IntegratorRTWStateStorageClass=Auto  FilterContinuousStateAttributes=''  FilterStateMustResolveToSignalObject=off  FilterRTWStateStorageClass=Auto  DifferentiatorICPrevScaledInput=0  DifferentiatorOutMin=[]  DifferentiatorOutMax=[]  InitialConditionSetting=State (most efficient)
      settings: LockScale=on
  Sum : Sum  Inputs=|+-
  Sum1 : Sum  Inputs=|+-
  Sum2 : Sum  Inputs=|+-
  u1 : Outport
  u2 : Outport  Port=2
  u3 : Outport  Port=3
  wires:
  vxd/1 -> Sum/1
  vz/1 -> Sum2/2
  vyd/1 -> Sum1/1
  vzd/1 -> Sum2/1
  vx/1 -> Sum/2
  "vy "/1 -> Sum1/2
  Sum/1 -> PID Controller/1
  PID Controller/1 -> u1/1
  Sum2/1 -> PID Controller2/1
  PID Controller2/1 -> u3/1
  PID Controller1/1 -> u2/1
  Sum1/1 -> PID Controller1/1

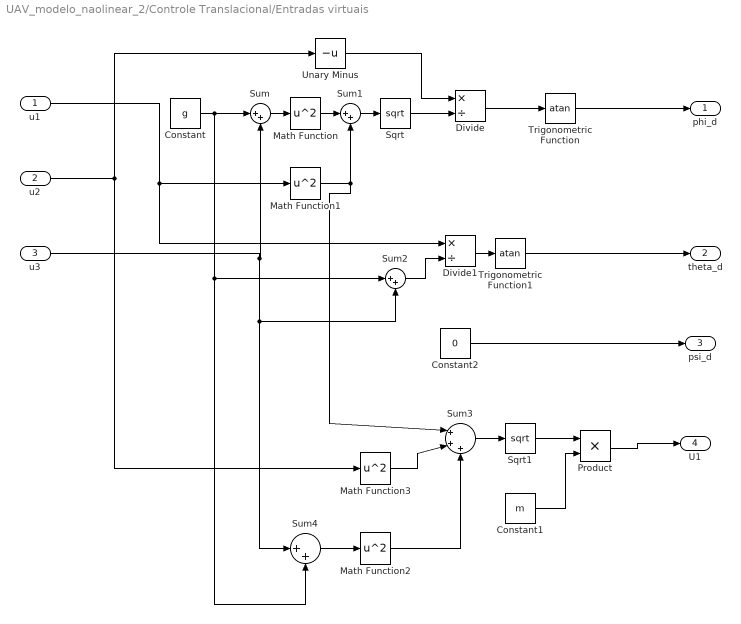
== system UAV_modelo_naolinear_2/Controle Translacional/Entradas virtuais ==
  u1 : Inport
  u2 : Inport  Port=2
  u3 : Inport  Port=3
  Constant : Constant  Value=g
  Constant1 : Constant  Value=m
  Constant2 : Constant  Value=0
  Divide : Product  Inputs=*/
  Divide1 : Product  Inputs=*/
  Math Function{,1..3} (4 alike) : Math  Operator=square  SaturateOnIntegerOverflow=on
  Product : Product
  Sqrt : Sqrt  SaturateOnIntegerOverflow=on
  Sqrt1 : Sqrt  SaturateOnIntegerOverflow=on
  Sum{,1..2,4} (4 alike) : Sum  Inputs=|++
  Sum3 : Sum  Inputs=|+++
  Trigonometric Function : Trigonometry  Operator=atan
  Trigonometric Function1 : Trigonometry  Operator=atan
  Unary Minus : UnaryMinus
  phi_d : Outport
  theta_d : Outport  Port=2
  psi_d : Outport  Port=3
  U1 : Outport  Port=4
  wires:
  Divide/1 -> Trigonometric Function/1
  Sqrt/1 -> Divide/2
  Trigonometric Function1/1 -> theta_d/1
  Sum1/1 -> Sqrt/1
  Divide1/1 -> Trigonometric Function1/1
  Sum/1 -> Math Function/1
  u1/1 -> Divide1/1, Math Function1/1
  Trigonometric Function/1 -> phi_d/1
  Sum2/1 -> Divide1/2
  Constant1/1 -> Product/2
  Math Function3/1 -> Sum3/2
  u2/1 -> Math Function3/1, Unary Minus/1
  Constant2/1 -> psi_d/1
  Sqrt1/1 -> Product/1
  Sum3/1 -> Sqrt1/1
  Math Function2/1 -> Sum3/3
  u3/1 -> Sum4/1, Sum2/2, Sum/2
  Constant/1 -> Sum4/2, Sum2/1, Sum/1
  Math Function/1 -> Sum1/1
  Product/1 -> U1/1
  Math Function1/1 -> Sum3/1, Sum1/2
  Sum4/1 -> Math Function2/1
  Unary Minus/1 -> Divide/1

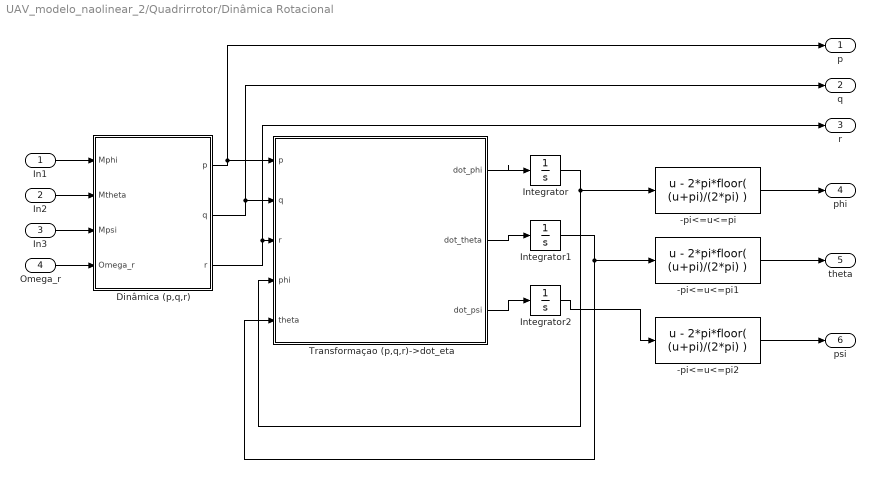
== system UAV_modelo_naolinear_2/Quadrirrotor/Dinâmica Rotacional ==
  In1 : Inport
  In2 : Inport  Port=2
  In3 : Inport  Port=3
  Omega_r : Inport  Port=4
  -pi<=u<=pi : Fcn  Expr=u - 2*pi*floor( (u+pi)/(2*pi) )
  -pi<=u<=pi1 : Fcn  Expr=u - 2*pi*floor( (u+pi)/(2*pi) )
  -pi<=u<=pi2 : Fcn  Expr=u - 2*pi*floor( (u+pi)/(2*pi) )
  Dinâmica (p,q,r) : Subsystem
      mask Display:
      | disp('(p,q,r)')
      | port_label('input',1,'Mphi')
      | port_label('input',2,'Mtheta')
      | port_label('input',3,'Mpsi')
      | port_label('input',4,'Omega_r')
      | port_label('output',1,'p')
      | port_label('output',2,'q')
      | port_label('output',3,'r')
  Integrator : Integrator  InitialCondition=phi0
  Integrator1 : Integrator  InitialCondition=theta0
  Integrator2 : Integrator  InitialCondition=psi0
  Transformaçao (p,q,r)->dot_eta : Subsystem  mask(output){}
      mask Display:
      | disp('dot_eta=f(eta,omega)')
      | port_label('input',1,'p')
      | port_label('input',2,'q')
      | port_label('input',3,'r')
      | port_label('input',4,'phi')
      | port_label('input',5,'theta')
      | port_label('output',1,'dot_phi')
      | port_label('output',2,'dot_theta')
      | port_label('output',3,'dot_psi')
  p : Outport
  q : Outport  Port=2
  r : Outport  Port=3
  phi : Outport  Port=4
  theta : Outport  Port=5
  psi : Outport  Port=6
  wires:
  Transformaçao (p,q,r)->dot_eta/2(dot_theta) -> Integrator1/1
  In3/1 -> Dinâmica (p,q,r)/3(Mpsi)
  Integrator1/1 -> -pi<=u<=pi1/1, Transformaçao (p,q,r)->dot_eta/5(theta)
  Integrator/1 -> -pi<=u<=pi/1, Transformaçao (p,q,r)->dot_eta/4(phi)
  In2/1 -> Dinâmica (p,q,r)/2(Mtheta)
  Transformaçao (p,q,r)->dot_eta/1(dot_phi) -> Integrator/1
  Transformaçao (p,q,r)->dot_eta/3(dot_psi) -> Integrator2/1
  Integrator2/1 -> -pi<=u<=pi2/1
  Dinâmica (p,q,r)/3(r) -> r/1, Transformaçao (p,q,r)->dot_eta/3(r)
  Dinâmica (p,q,r)/2(q) -> q/1, Transformaçao (p,q,r)->dot_eta/2(q)
  Dinâmica (p,q,r)/1(p) -> p/1, Transformaçao (p,q,r)->dot_eta/1(p)
  In1/1 -> Dinâmica (p,q,r)/1(Mphi)
  -pi<=u<=pi/1 -> phi/1
  -pi<=u<=pi1/1 -> theta/1
  -pi<=u<=pi2/1 -> psi/1
  Omega_r/1 -> Dinâmica (p,q,r)/4(Omega_r)

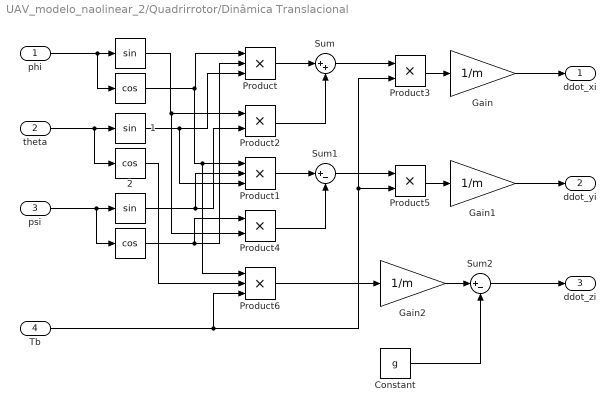
== system UAV_modelo_naolinear_2/Quadrirrotor/Dinâmica Translacional ==
  phi : Inport
  theta : Inport  Port=2
  psi : Inport  Port=3
  Tb : Inport  Port=4
  " " : Trigonometry
  "  " : Trigonometry  Operator=cos
  "   " : Trigonometry  Operator=cos
  "    " : Trigonometry  Operator=cos
  " 1" : Trigonometry
  " 2" : Trigonometry
  Constant : Constant  Value=g
  Gain : Gain  Gain=1/m
  Gain1 : Gain  Gain=1/m
  Gain2 : Gain  Gain=1/m
  Product : Product  Inputs=3
  Product1 : Product  Inputs=3
  Product{2..5} (4 alike) : Product
  Product6 : Product  Inputs=3
  Sum : Sum  Inputs=|++
  Sum1 : Sum  Inputs=|+-
  Sum2 : Sum  Inputs=|+-
  ddot_xi : Outport
  ddot_yi : Outport  Port=2
  ddot_zi : Outport  Port=3
  wires:
  Product6/1 -> Gain2/1
  Product3/1 -> Gain/1
  Sum2/1 -> ddot_zi/1
  " 1"/1 -> Product1/3, Product/3
  Product1/1 -> Sum1/1
  phi/1 -> "  "/1, " "/1
  " 2"/1 -> Product1/2, Product2/2
  "    "/1 -> Product4/1, Product/2
  Sum/1 -> Product3/1
  Product2/1 -> Sum/2
  " "/1 -> Product4/2, Product2/1
  Constant/1 -> Sum2/2
  Gain1/1 -> ddot_yi/1
  theta/1 -> "   "/1, " 1"/1
  Product5/1 -> Gain1/1
  psi/1 -> "    "/1, " 2"/1
  Tb/1 -> Product5/2, Product3/2, Product6/3
  Product/1 -> Sum/1
  Product4/1 -> Sum1/2
  Gain2/1 -> Sum2/1
  "   "/1 -> Product6/2
  "  "/1 -> Product6/1, Product1/1, Product/1
  Gain/1 -> ddot_xi/1
  Sum1/1 -> Product5/1

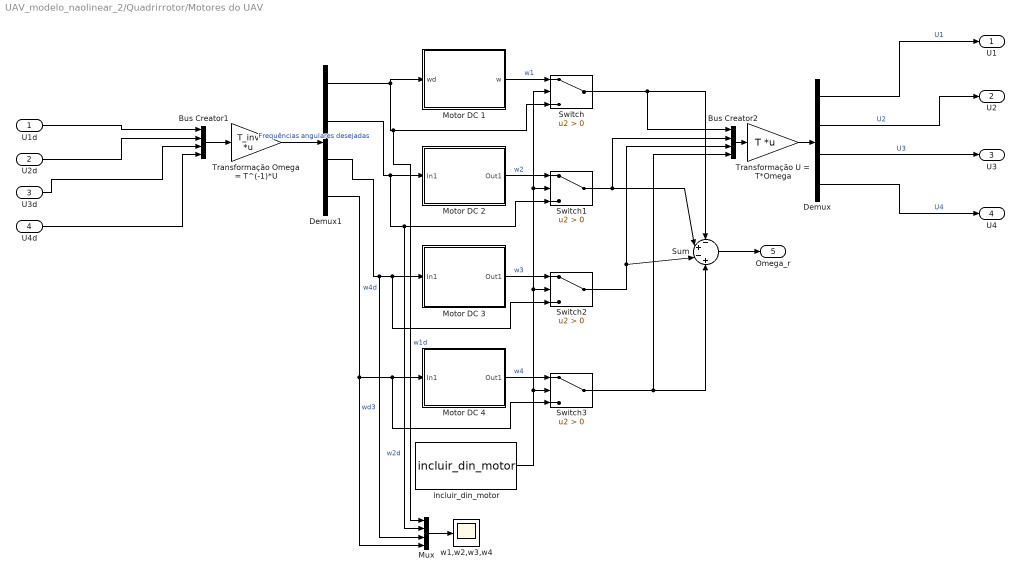
== system UAV_modelo_naolinear_2/Quadrirrotor/Motores do UAV  ==
  U1d : Inport
  U2d : Inport  Port=2
  U3d : Inport  Port=3
  U4d : Inport  Port=4
  Bus Creator1 : BusCreator  Inputs=4
  Bus Creator2 : BusCreator  Inputs=4
  Demux : Demux
  Demux1 : Demux
  Motor DC 1 : Subsystem
      mask Display:
      | disp('Motor DC')
      | port_label('input',1,'wd')
      | port_label('output',1,'w')
  Motor DC 2 : Subsystem
      mask Display:
      | disp('Motod DC')
      | port_label('input',1,'wd')
      | port_label('output',1,'w')
  Motor DC 3 : Subsystem
      mask Display:
      | disp('Motod DC')
      | port_label('input',1,'wd')
      | port_label('output',1,'w')
  Motor DC 4 : Subsystem
      mask Display:
      | disp('Motod DC')
      | port_label('input',1,'wd')
      | port_label('output',1,'w')
  Mux : Mux
  Sum : Sum  Inputs=-+-+
  Switch{,1..3} (4 alike) : Switch  Criteria=u2 > Threshold
  Transformação Omega = T^(-1)*U : Gain  Gain=T_inv  Multiplication=Matrix(K*u)  RndMeth=Nearest  LockScale=on
  Transformação U = T*Omega : Gain  Gain=T  Multiplication=Matrix(K*u)  RndMeth=Nearest  LockScale=on
  incluir_din_motor : Constant  Value=incluir_din_motor
  w1,w2,w3,w4 : Scope
  U1 : Outport
  U2 : Outport  Port=2
  U3 : Outport  Port=3
  U4 : Outport  Port=4
  Omega_r : Outport  Port=5
  wires:
  Demux1/1 -> Motor DC 1/1(wd), Mux/1, Switch/3  "w1d"
  Bus Creator2/1 -> Transformação U = T*Omega/1
  Transformação Omega = T^(-1)*U/1 -> Demux1/1  "Frequências angulares desejadas"
  Transformação U = T*Omega/1 -> Demux/1
  Demux/4 -> U4/1  "U4"
  Demux/3 -> U3/1  "U3"
  Bus Creator1/1 -> Transformação Omega = T^(-1)*U/1
  Demux/2 -> U2/1  "U2"
  Demux/1 -> U1/1  "U1"
  Sum/1 -> Omega_r/1
  Demux1/2 -> Mux/2, Switch1/3, Motor DC 2/1(In1)  "w2d"
  Demux1/3 -> Mux/3, Switch2/3, Motor DC 3/1(In1)  "wd3"
  Demux1/4 -> Mux/4, Switch3/3, Motor DC 4/1(In1)  "w4d"
  Switch/1 -> Sum/1, Bus Creator2/1
  Motor DC 1/1(w) -> Switch/1  "w1"
  Motor DC 2/1(Out1) -> Switch1/1  "w2"
  Switch1/1 -> Sum/2, Bus Creator2/2
  Motor DC 3/1(Out1) -> Switch2/1  "w3"
  Switch2/1 -> Sum/3, Bus Creator2/3
  Motor DC 4/1(Out1) -> Switch3/1  "w4"
  Switch3/1 -> Sum/4, Bus Creator2/4
  incluir_din_motor/1 -> Switch/2, Switch1/2, Switch2/2, Switch3/2
  Mux/1 -> w1,w2,w3,w4/1
  U1d/1 -> Bus Creator1/1
  U2d/1 -> Bus Creator1/2
  U3d/1 -> Bus Creator1/3
  U4d/1 -> Bus Creator1/4

== system UAV_modelo_naolinear_2/Quadrirrotor/Dinâmica Rotacional/Dinâmica (p,q,r) ==
  Mphi : Inport
  Mtheta : Inport  Port=2
  Mpsi : Inport  Port=3
  Omega_r : Inport  Port=4
  "  " : Subsystem
      mask Display:
      | disp('Dinâmica Rotacional no Corpo')
      | port_label('input',1,'p')
      | port_label('input',2,'q')
      | port_label('input',3,'r')
      | port_label('input',4,'Mphi')
      | port_label('input',5,'Mtheta')
      | port_label('input',6,'Mpsi')
      | port_label('input',7,'Omega_r')
      | port_label('output',1,'dot_p')
      | port_label('output',2,'dot_q')
      | port_label('output',3,'dot_r')
  Integrator : Integrator  InitialCondition=p0
  Integrator1 : Integrator  InitialCondition=q0
  Integrator2 : Integrator  InitialCondition=r0
  p : Outport
  q : Outport  Port=2
  r : Outport  Port=3
  wires:
  "  "/3(dot_r) -> Integrator2/1
  Integrator2/1 -> r/1, "  "/3(r)
  "  "/2(dot_q) -> Integrator1/1
  "  "/1(dot_p) -> Integrator/1
  Integrator1/1 -> q/1, "  "/2(q)
  Integrator/1 -> p/1, "  "/1(p)
  Mpsi/1 -> "  "/6(Mpsi)
  Mtheta/1 -> "  "/5(Mtheta)
  Mphi/1 -> "  "/4(Mphi)
  Omega_r/1 -> "  "/7(Omega_r)

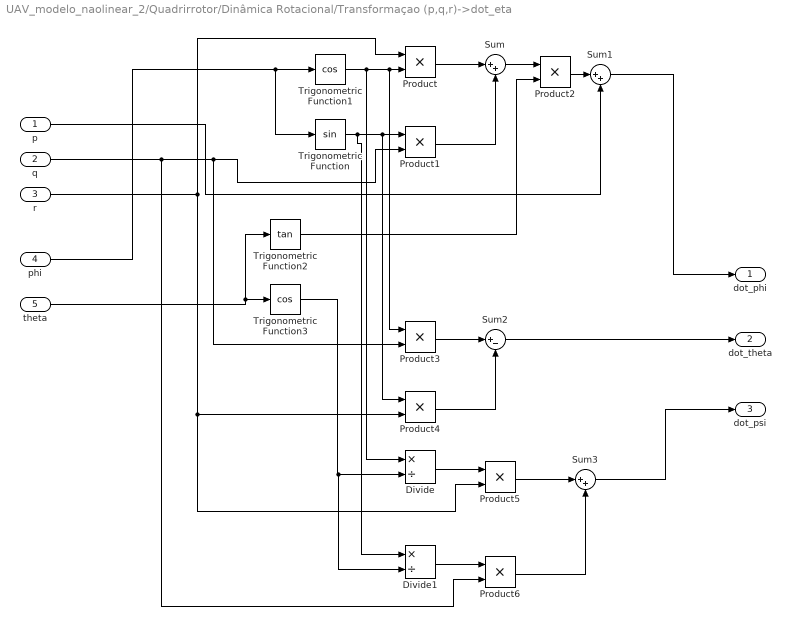
== system UAV_modelo_naolinear_2/Quadrirrotor/Dinâmica Rotacional/Transformaçao (p,q,r)->dot_eta ==
  p : Inport
  q : Inport  Port=2
  r : Inport  Port=3
  phi : Inport  Port=4
  theta : Inport  Port=5
  Divide : Product  Inputs=*/
  Divide1 : Product  Inputs=*/
  Product{,1..6} (7 alike) : Product
  Sum : Sum  Inputs=|++
  Sum1 : Sum  Inputs=|++
  Sum2 : Sum  Inputs=|+-
  Sum3 : Sum  Inputs=|++
  Trigonometric Function : Trigonometry
  Trigonometric Function1 : Trigonometry  Operator=cos
  Trigonometric Function2 : Trigonometry  Operator=tan
  Trigonometric Function3 : Trigonometry  Operator=cos
  dot_phi : Outport
  dot_theta : Outport  Port=2
  dot_psi : Outport  Port=3
  wires:
  Sum1/1 -> dot_phi/1
  Sum2/1 -> dot_theta/1
  Sum3/1 -> dot_psi/1
  Trigonometric Function/1 -> Divide1/1, Product4/1, Product1/1
  Product/1 -> Sum/1
  r/1 -> Product5/2, Product4/2, Product/1
  q/1 -> Product6/2, Product3/2, Product1/2
  Product1/1 -> Sum/2
  phi/1 -> Trigonometric Function/1, Trigonometric Function1/1
  Trigonometric Function2/1 -> Product2/2
  Sum/1 -> Product2/1
  Product2/1 -> Sum1/1
  p/1 -> Sum1/2
  Trigonometric Function1/1 -> Divide/1, Product3/1, Product/2
  Product3/1 -> Sum2/1
  Product4/1 -> Sum2/2
  Divide/1 -> Product5/1
  Product5/1 -> Sum3/1
  Divide1/1 -> Product6/1
  Product6/1 -> Sum3/2
  theta/1 -> Trigonometric Function2/1, Trigonometric Function3/1
  Trigonometric Function3/1 -> Divide1/2, Divide/2

== system UAV_modelo_naolinear_2/Quadrirrotor/Motores do UAV /Motor DC 1 ==
  wd : Inport
  Modelo Motor 1 : TransferFcn  Numerator=[Kp]  Denominator=[tau_a 1]
  Transport Delay : TransportDelay  DelayTime=tau_s  PadeOrder=2
  w : Outport
  wires:
  Modelo Motor 1/1 -> Transport Delay/1
  Transport Delay/1 -> w/1  "w1"
  wd/1 -> Modelo Motor 1/1

== system UAV_modelo_naolinear_2/Quadrirrotor/Motores do UAV /Motor DC 2 ==
  In1 : Inport
  Modelo Motor 2 : TransferFcn  Numerator=[Kp]  Denominator=[tau_a 1]
  Transport Delay1 : TransportDelay  DelayTime=tau_s  PadeOrder=2
  Out1 : Outport
  wires:
  Modelo Motor 2/1 -> Transport Delay1/1
  In1/1 -> Modelo Motor 2/1
  Transport Delay1/1 -> Out1/1  "w2"

== system UAV_modelo_naolinear_2/Quadrirrotor/Motores do UAV /Motor DC 3 ==
  In1 : Inport
  Modelo Motor 3 : TransferFcn  Numerator=[Kp]  Denominator=[tau_a 1]
  Transport Delay2 : TransportDelay  DelayTime=tau_s  PadeOrder=2
  Out1 : Outport
  wires:
  In1/1 -> Modelo Motor 3/1
  Modelo Motor 3/1 -> Transport Delay2/1
  Transport Delay2/1 -> Out1/1  "w3"

== system UAV_modelo_naolinear_2/Quadrirrotor/Motores do UAV /Motor DC 4 ==
  In1 : Inport
  Modelo Motor 4 : TransferFcn  Numerator=[Kp]  Denominator=[tau_a 1]
  Transport Delay3 : TransportDelay  DelayTime=tau_s  PadeOrder=2
  Out1 : Outport
  wires:
  Modelo Motor 4/1 -> Transport Delay3/1
  In1/1 -> Modelo Motor 4/1
  Transport Delay3/1 -> Out1/1  "w4"

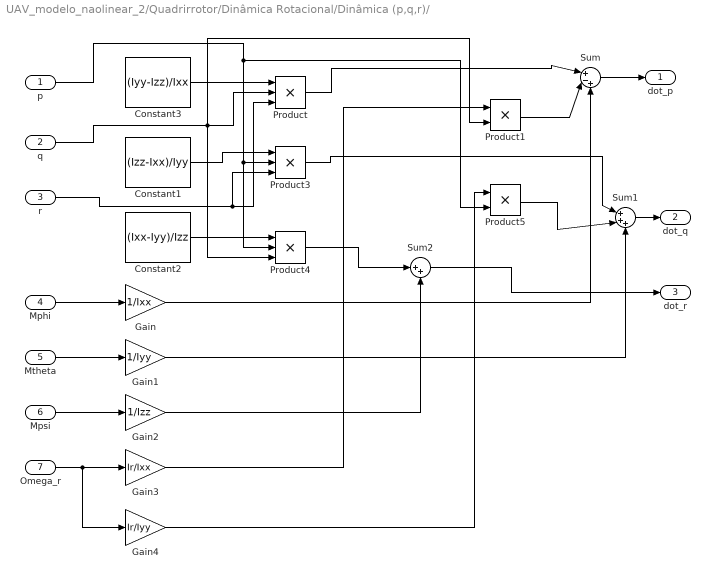
== system UAV_modelo_naolinear_2/Quadrirrotor/Dinâmica Rotacional/Dinâmica (p,q,r)/   ==
  p : Inport
  q : Inport  Port=2
  r : Inport  Port=3
  Mphi : Inport  Port=4
  Mtheta : Inport  Port=5
  Mpsi : Inport  Port=6
  Omega_r : Inport  Port=7
  Constant1 : Constant  Value=(Izz-Ixx)/Iyy
  Constant2 : Constant  Value=(Ixx-Iyy)/Izz
  Constant3 : Constant  Value=(Iyy-Izz)/Ixx
  Gain : Gain  Gain=1/Ixx
  Gain1 : Gain  Gain=1/Iyy
  Gain2 : Gain  Gain=1/Izz
  Gain3 : Gain  Gain=Ir/Ixx
  Gain4 : Gain  Gain=Ir/Iyy
  Product : Product  Inputs=3
  Product1 : Product
  Product3 : Product  Inputs=3
  Product4 : Product  Inputs=3
  Product5 : Product
  Sum : Sum  Inputs=|+-+
  Sum1 : Sum  Inputs=|+++
  Sum2 : Sum  Inputs=|++
  dot_p : Outport
  dot_q : Outport  Port=2
  dot_r : Outport  Port=3
  wires:
  Product/1 -> Sum/1
  Sum/1 -> dot_p/1
  Constant1/1 -> Product3/1
  Constant3/1 -> Product/1
  r/1 -> Product3/3, Product/3
  Gain1/1 -> Sum1/3
  Mtheta/1 -> Gain1/1
  p/1 -> Product5/2, Product4/2, Product3/2
  Gain/1 -> Sum/3
  q/1 -> Product4/3, Product1/2, Product/2
  Product4/1 -> Sum2/1
  Mpsi/1 -> Gain2/1
  Constant2/1 -> Product4/1
  Sum2/1 -> dot_r/1
  Gain4/1 -> Product5/1
  Product1/1 -> Sum/2
  Product3/1 -> Sum1/1
  Gain2/1 -> Sum2/2
  Gain3/1 -> Product1/1
  Product5/1 -> Sum1/2
  Mphi/1 -> Gain/1
  Sum1/1 -> dot_q/1
  Omega_r/1 -> Gain4/1, Gain3/1
